simulink model "final_intelligent_adaptive_modulation_selector_using_BER"  (R2025b)
settings: Solver=VariableStepAuto  StartTime=0.0  StopTime=5000  RelTol=1e-3
libraries: commchan3 x5, commdigbbndpm3 x4, commsink2 x4, simulink x2, commdigbbndfm2 x2, commdigbbndam3 x2, commrandsrc3 x1
settings Model: Creator=nimma  LastModifiedBy=nimma

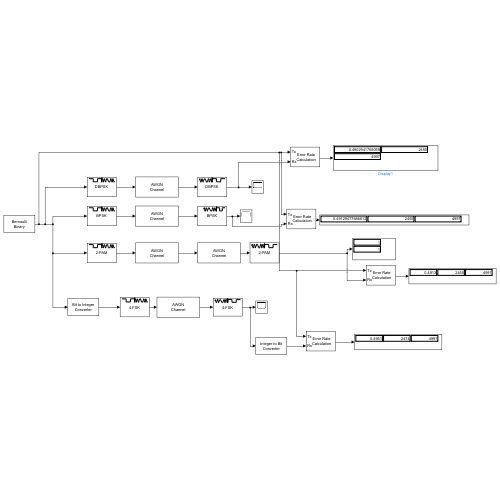
[thumbnail: Simulink's stored preview of the top-level diagram]
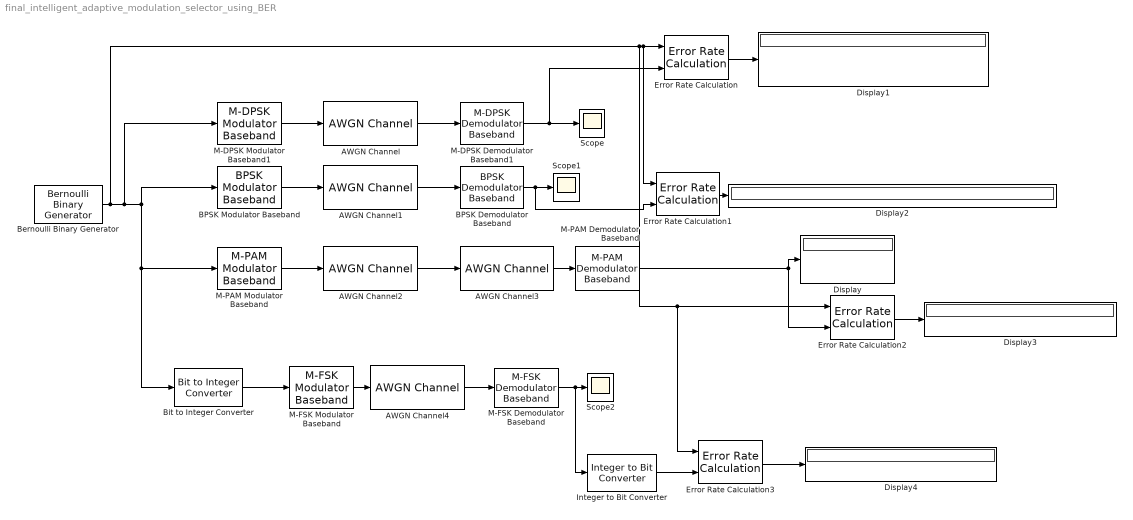
== system final_intelligent_adaptive_modulation_selector_using_BER ==
  AWGN Channel{,1..2,4} (4 alike) : commchan3/AWGN Channel  LegacyMode=off  NoiseMethod="Signal to noise ratio  (Eb/No)"  noiseMode="Signal to noise ratio  (SNR)"  EbNo=8  EsNo=10  SNR=10  BitsPerSymbol=1  SignalPower=1  SpecifySymbolPeriod=off  SamplesPerSymbol=1  SymbolPeriod=1  VarianceSource=Parameter  Variance=1  RandomStream=Global stream  Seed=67  SimulateUsing=Code generation
  AWGN Channel3 : commchan3/AWGN Channel  LegacyMode=off  NoiseMethod="Signal to noise ratio  (SNR)"  noiseMode="Signal to noise ratio  (SNR)"  EbNo=10  EsNo=10  SNR=10  BitsPerSymbol=1  SignalPower=1  SpecifySymbolPeriod=off  SamplesPerSymbol=1  SymbolPeriod=1  VarianceSource=Parameter  Variance=1  RandomStream=Global stream  Seed=67  SimulateUsing=Code generation
  BPSK Demodulator Baseband : commdigbbndpm3/BPSK Demodulator Baseband  DecType=Hard decision  VarSource=Dialog  Variance=1  Ph=0  outDtype=Inherit via internal rule  derotateFactorWordLen=16  derotateFactorDataTypeStr=Inherit: Same word length as input  derotateFactorLastDataTypeStr=Inherit: Same word length as input
  BPSK Modulator Baseband : commdigbbndpm3/BPSK Modulator Baseband  Ph=0  outDtype=double  outWordLen=16  outUDDataType=sfix(16)  outFracLenMode=Best precision  outFracLen=15  outDataTypeStr=double  outLastDataTypeStr=double
  Bernoulli Binary Generator : commrandsrc3/Bernoulli Binary Generator  ProbabilityOfZero=0.5  SeedSource=Auto  Seed=0  SampleTime=1  SamplesPerFrame=2  OutputDataType=double  SimulateUsing=Interpreted execution
  Bit to Integer Converter : simulink/Logic and Bit Operations/Bit to Integer Converter  nbits=2  bitOrder=MSB first  signedOutputValues=Unsigned  outDtype=Smallest integer  outDtypeSigned=Inherit via internal rule
  Display{,1..4} (5 alike) : Display
  Error Rate Calculation{,1..3} (4 alike) : commsink2/Error Rate Calculation  N=5  st_delay=0  cp_mode=Entire frame  subframe=[]  PMode=Port  WsName=ErrorVec  RsMode2=off  stop=off  numErr=100  maxBits=1e6
  Integer to Bit Converter : simulink/Logic and Bit Operations/Integer to Bit Converter  nbits=2  signedInputValues=Unsigned  bitOrder=MSB first  outDtype=double
  M-DPSK Demodulator Baseband1 : commdigbbndpm3/M-DPSK Demodulator Baseband  M=2  OutType=Integer  Dec=Gray  Ph=0  outDtype1=Inherit via internal rule  outDtype2=Inherit via internal rule
  M-DPSK Modulator Baseband1 : commdigbbndpm3/M-DPSK Modulator Baseband  M=2  InType=Integer  Enc=Gray  Ph=0  outDtype=double
  M-FSK Demodulator Baseband : commdigbbndfm2/M-FSK Demodulator Baseband  M=4  OutType=Integer  Dec=Gray  freqSep=500  numSamp=8  RateOptions=Enforce single-rate processing  outDataType=double
  M-FSK Modulator Baseband : commdigbbndfm2/M-FSK Modulator Baseband  M=4  InType=Integer  Enc=Gray  freqSep=500  phaseType=Continuous  numSamp=8  RateOptions=Enforce single-rate processing  outDataType=double
  M-PAM Demodulator Baseband : commdigbbndam3/M-PAM Demodulator Baseband  M=2  OutType=Integer  Dec=Gray  PowType=Min. distance between symbols  MinDist=2  AvgPow=1  PeakPow=1  outDtype1=Inherit via internal rule  outDtype2=Inherit via internal rule  denormFactorWordLen=16  denormFactorDataTypeStr=Inherit: Same word length as input  denormFactorLastDataTypeStr=Inherit: Same word length as input  prodOutWordLen=16  prodOutRoundingMode=Floor  prodOutOverflowMode=Wrap  prodOutOvFlMode=off  prodOutOvFlModeLastStrValue=off  sumWordLen=16
  M-PAM Modulator Baseband : commdigbbndam3/M-PAM Modulator Baseband  M=2  InType=Integer  Enc=Gray  PowType=Min. distance between symbols  MinDist=2  AvgPow=1  PeakPow=1  outDtype=double  outWordLen=16  outUDDataType=sfix(16)  outFracLenMode=Best precision  outFracLen=15  outDataTypeStr=double  outLastDataTypeStr=double
  Scope : Scope
      settings: ActiveDisplayYMinimum=-0.12499999999999997  ActiveDisplayYMaximum=1.125
  Scope1 : Scope
      settings: ActiveDisplayYMinimum=-0.31992275527366565  ActiveDisplayYMaximum=1.1994600572263348
  Scope2 : Scope
      settings: ActiveDisplayYMinimum=-1  ActiveDisplayYMaximum=1  DataLoggingVariableName=ScopeData2
  wires:
  Bernoulli Binary Generator/1 -> Error Rate Calculation2/1, Error Rate Calculation3/1, Error Rate Calculation1/1, Error Rate Calculation/1, M-DPSK Modulator Baseband1/1, BPSK Modulator Baseband/1, Bit to Integer Converter/1, M-PAM Modulator Baseband/1
  M-DPSK Modulator Baseband1/1 -> AWGN Channel/1
  BPSK Modulator Baseband/1 -> AWGN Channel1/1
  Bit to Integer Converter/1 -> M-FSK Modulator Baseband/1
  AWGN Channel/1 -> M-DPSK Demodulator Baseband1/1
  AWGN Channel1/1 -> BPSK Demodulator Baseband/1
  M-PAM Demodulator Baseband/1 -> Error Rate Calculation2/2, Display/1
  AWGN Channel2/1 -> AWGN Channel3/1
  BPSK Demodulator Baseband/1 -> Error Rate Calculation1/2, Scope1/1
  M-FSK Modulator Baseband/1 -> AWGN Channel4/1
  AWGN Channel4/1 -> M-FSK Demodulator Baseband/1
  M-FSK Demodulator Baseband/1 -> Integer to Bit Converter/1, Scope2/1
  Error Rate Calculation/1 -> Display1/1
  Error Rate Calculation1/1 -> Display2/1
  Error Rate Calculation2/1 -> Display3/1
  Integer to Bit Converter/1 -> Error Rate Calculation3/2
  Error Rate Calculation3/1 -> Display4/1
  M-DPSK Demodulator Baseband1/1 -> Error Rate Calculation/2, Scope/1
  M-PAM Modulator Baseband/1 -> AWGN Channel2/1
  AWGN Channel3/1 -> M-PAM Demodulator Baseband/1
